simulink model "power_supply_image"  (R2023b)
settings: Solver=ode1  StartTime=0.0  StopTime=time/3  FixedStep=1e-6  RelTol=1e-3
undefined symbols (not defined in the file or in its folder): C1, C2, D1, L1, L2
libraries: spsDiodeLib x13, spsIdealSwitchLib x8, spsVoltageMeasurementLib x6, spsSeriesRLCBranchLib x5, spsCurrentMeasurementLib x2, spsLinearTransformerLib x2, spsDCVoltageSourceLib x1, simulink x1, spspowerguiLib x1
settings Model: Creator=lyapunov  LastModifiedBy=lyapunov
settings OptimizationCC: ReuseModelBlockBuffer=off

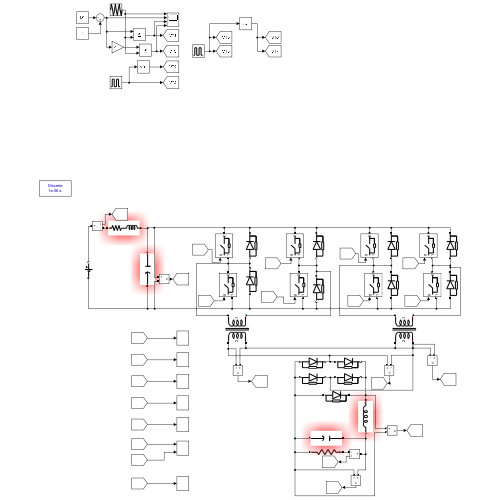
[thumbnail: Simulink's stored preview of the top-level diagram]
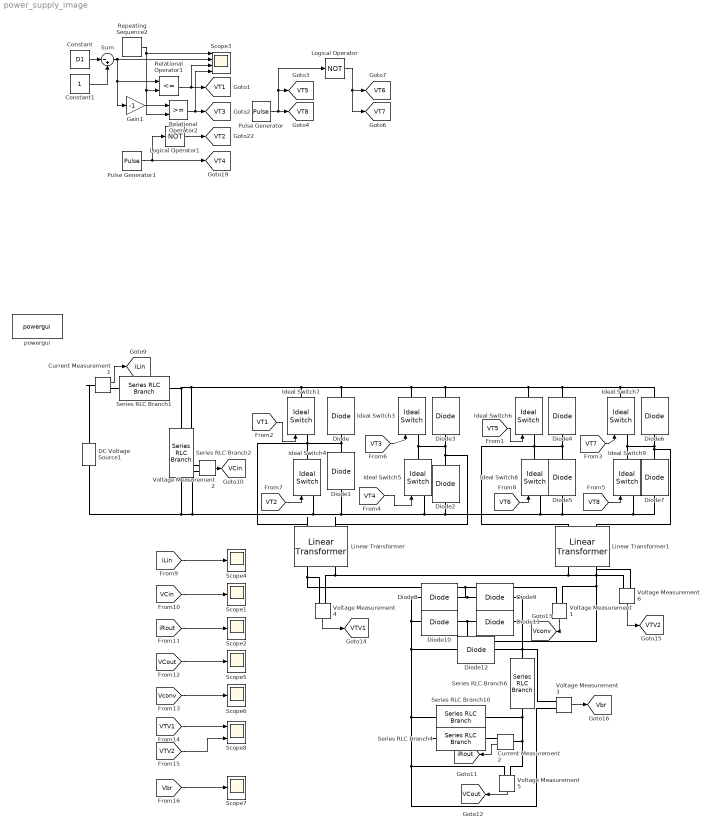
== system power_supply_image ==
  Constant : Constant  Value=D1
  Constant1 : Constant
  Current Measurement1 : spsCurrentMeasurementLib/Current Measurement  PhasorSimulation=off  OutputType=Complex  PSBequivalent=0
  Current Measurement2 : spsCurrentMeasurementLib/Current Measurement  PhasorSimulation=off  OutputType=Complex  PSBequivalent=0
  DC Voltage Source1 : spsDCVoltageSourceLib/DC Voltage Source  Amplitude=300  Measurements=None
  Diode{,1..12} (13 alike) : spsDiodeLib/Diode  Ron=0.001  Lon=0  Vf=0.8  IC=0  UseSnubber=0  Rs=5000  Cs=250e-9  Measurements=off
  Gain1 : Gain  Gain=-1
  Ideal Switch{1,3..9} (8 alike) : spsIdealSwitchLib/Ideal Switch  Ron=0.001  Lon=0  IC=0  Rs=1e5  Cs=inf  Measurements=off
  Linear Transformer : spsLinearTransformerLib/Linear Transformer  UNITS=SI  NominalPower=[500 10000 ]  winding1=[300 0 0]  winding2=[150 0 0]  ThreeWindings=off  winding3=[3.15e+05 0.7938 0.084225]  RmLm=[1e6 1e6]  Measurements=None  DataType=on
  Linear Transformer1 : spsLinearTransformerLib/Linear Transformer  UNITS=SI  NominalPower=[ 500 10000 ]  winding1=[300 0 0]  winding2=[150 0 0]  ThreeWindings=off  winding3=[3.15e+05 0.7938 0.084225]  RmLm=[1e6 1e6]  Measurements=None  DataType=on
  Logical Operator : Logic  Operator=NOT  AllPortsSameDT=off  OutDataTypeStr=boolean
  Logical Operator1 : Logic  Operator=NOT  AllPortsSameDT=off  OutDataTypeStr=boolean
  Pulse Generator : DiscretePulseGenerator  PulseType=Time based  Period=1/10000  PulseWidth=50
  Pulse Generator1 : DiscretePulseGenerator  PulseType=Time based  Period=1/10000  PulseWidth=50
  Relational Operator1 : RelationalOperator  Operator=<=  OutDataTypeStr=boolean  RndMeth=Simplest  InputSameDT=off
  Relational Operator2 : RelationalOperator  OutDataTypeStr=boolean  RndMeth=Simplest  InputSameDT=off
  Repeating Sequence2 : simulink/Sources/Repeating Sequence  rep_seq_t=[0 0.5/20000 1/20000 1.5/20000 2/20000]  rep_seq_y=[0 1 0 -1 0]
  Scope{1..2,4..7} (6 alike) : Scope
  Scope3 : Scope  NumInputPorts=4
  Scope8 : Scope  NumInputPorts=2
  Series RLC Branch1 : spsSeriesRLCBranchLib/Series RLC Branch  LConnTagsString=__new0  RConnTagsString=__new0  BranchType=RL  Resistance=0.01  Inductance=L1  SetiL0=off  InitialCurrent=0  Capacitance=1e-6  Setx0=off  InitialVoltage=0  Measurements=None
  Series RLC Branch10 : spsSeriesRLCBranchLib/Series RLC Branch  LConnTagsString=__new0  RConnTagsString=__new0  BranchType=C  Resistance=1  Inductance=10e-3  SetiL0=off  InitialCurrent=0  Capacitance=C2  Setx0=off  InitialVoltage=0  Measurements=None
  Series RLC Branch2 : spsSeriesRLCBranchLib/Series RLC Branch  LConnTagsString=__new0  RConnTagsString=__new0  BranchType=C  Resistance=1  Inductance=10e-3  SetiL0=off  InitialCurrent=0  Capacitance=C1  Setx0=off  InitialVoltage=0  Measurements=None
  Series RLC Branch4 : spsSeriesRLCBranchLib/Series RLC Branch  LConnTagsString=__new0  RConnTagsString=__new0  BranchType=R  Resistance=87.23  Inductance=10e-3  SetiL0=off  InitialCurrent=0  Capacitance=100e-6  Setx0=off  InitialVoltage=0  Measurements=None
  Series RLC Branch6 : spsSeriesRLCBranchLib/Series RLC Branch  LConnTagsString=__new0  RConnTagsString=__new0  BranchType=L  Resistance=0.01  Inductance=L2  SetiL0=off  InitialCurrent=0  Capacitance=1e-6  Setx0=off  InitialVoltage=0  Measurements=None
  Sum : Sum  Inputs=|-+
  Voltage Measurement{1..6} (6 alike) : spsVoltageMeasurementLib/Voltage Measurement  PhasorSimulation=off  OutputType=Complex  PSBequivalent=0
  powergui : spspowerguiLib/powergui  Priority=1  SimulationMode=Discrete  SampleTime=1e-6  frequency=60  Iterations=50  frequencyindice=0  Pbase=100e6  ErrMax=1e-4  UnitsV=kV  UnitsW=MW  buscounter=0  FunctionMessages=off  echomessages=off  EnableUseOfTLC=off  CurrentSourceSwitches=off  DisableSnubberDevices=off  DisableRonSwitches=off  DisableVfSwitches=off  DisplayEquations=off  AutomaticDiscreteSolvers=off  SolverType=Tustin/Backward Euler (TBE)  Interpol=off  ExternalGateDelay=off  methode=off  Ts=100  x0status=zero  SPID=on  SwTol=0  HookPort=off  NonlinearTolerance=1e-4  nMaxIteration=100  ContinueOnMaxIteration=off  RestoreLinks=warning  ResistiveCurrentMeasurement=off  Frange=[0:2:500]  Ylog=off  Xlog=on  ShowGrid=off  save=off  variable=ZData  structure=0  ZoomFFT=off  StartTime=0.0  cycles=1  DisplayStyle=1  fundamental=60  FreqAxis=off  MaxFrequency=1000  frequencyindicesteady=1  RmsSteady=1  display=off
  tag scope: VCin=global, VCout=global, VT1=global, VT2=global, VT3=global, VT4=global, VT5=global, VT6=global, VT7=global, VT8=global, VTV1=global, VTV2=global, Vbr=global, Vconv=global, iLin=global, iRout=global
  wires:
  Pulse Generator/1 -> Logical Operator/1, [VT5], [VT8]
  Logical Operator/1 -> [VT7], [VT6]
  Repeating Sequence2/1 -> Relational Operator1/2, Relational Operator2/2, Scope3/1
  Relational Operator1/1 -> [VT1], Scope3/3
  Sum/1 -> Relational Operator1/1, Gain1/1, Scope3/2
  Relational Operator2/1 -> [VT3], Scope3/4
  Gain1/1 -> Relational Operator2/1
  [VT5] -> Ideal Switch6/1
  [VT7] -> Ideal Switch7/1
  Constant/1 -> Sum/1
  Constant1/1 -> Sum/2
  Voltage Measurement1/1 -> [Vconv]
  Voltage Measurement2/1 -> [VCin]
  [VT8] -> Ideal Switch9/1
  [VT4] -> Ideal Switch5/1
  [VT1] -> Ideal Switch1/1
  [VT3] -> Ideal Switch3/1
  [VT2] -> Ideal Switch4/1
  [VT6] -> Ideal Switch8/1
  Current Measurement1/1 -> [iLin]
  Current Measurement2/1 -> [iRout]
  Voltage Measurement5/1 -> [VCout]
  [iLin] -> Scope4/1
  [VCin] -> Scope1/1
  [iRout] -> Scope2/1
  [VCout] -> Scope5/1
  [Vconv] -> Scope6/1
  Voltage Measurement3/1 -> [Vbr]
  Voltage Measurement4/1 -> [VTV1]
  Voltage Measurement6/1 -> [VTV2]
  [VTV1] -> Scope8/1
  [VTV2] -> Scope8/2
  [Vbr] -> Scope7/1
  Logical Operator1/1 -> [VT2]
  Pulse Generator1/1 -> Logical Operator1/1, [VT4]
  connections:
  Current Measurement1/RConn1 -- Series RLC Branch1/LConn1
  Current Measurement1/LConn1 -- DC Voltage Source1/RConn1
  Ideal Switch5/RConn1 -- Linear Transformer/LConn1 -- Diode2/RConn1 -- Diode3/LConn1 -- Ideal Switch3/LConn1
  Ideal Switch6/LConn1 -- Ideal Switch8/RConn1 -- Linear Transformer1/LConn2 -- Diode5/RConn1 -- Diode4/LConn1
  Ideal Switch5/LConn1 -- Diode2/LConn1 -- Diode7/LConn1 -- Ideal Switch9/LConn1 -- Diode5/LConn1 -- Ideal Switch8/LConn1 -- Diode1/LConn1 -- DC Voltage Source1/LConn1 -- Series RLC Branch2/RConn1 -- Voltage Measurement2/LConn2 -- Ideal Switch4/LConn1
  Ideal Switch1/LConn1 -- Ideal Switch4/RConn1 -- Linear Transformer/LConn2 -- Diode/LConn1 -- Diode1/RConn1
  Ideal Switch9/RConn1 -- Diode7/RConn1 -- Linear Transformer1/LConn1 -- Diode6/LConn1 -- Ideal Switch7/LConn1
  Diode8/RConn1 -- Voltage Measurement4/LConn2 -- Linear Transformer/RConn2 -- Voltage Measurement1/LConn1 -- Diode9/LConn1
  Linear Transformer1/RConn1 -- Voltage Measurement6/LConn1 -- Diode10/RConn1 -- Diode11/LConn1 -- Voltage Measurement1/LConn2
  Series RLC Branch4/RConn1 -- Voltage Measurement5/LConn2 -- Voltage Measurement3/LConn2 -- Diode12/LConn1 -- Diode8/LConn1 -- Diode10/LConn1 -- Series RLC Branch10/RConn1
  Diode9/RConn1 -- Series RLC Branch6/LConn1 -- Voltage Measurement3/LConn1 -- Diode12/RConn1 -- Diode11/RConn1
  Series RLC Branch10/LConn1 -- Current Measurement2/LConn1 -- Voltage Measurement5/LConn1 -- Series RLC Branch6/RConn1
  Diode4/RConn1 -- Series RLC Branch1/RConn1 -- Series RLC Branch2/LConn1 -- Voltage Measurement2/LConn1 -- Ideal Switch1/RConn1 -- Diode/RConn1 -- Ideal Switch3/RConn1 -- Diode3/RConn1 -- Ideal Switch6/RConn1 -- Diode6/RConn1 -- Ideal Switch7/RConn1
  Current Measurement2/RConn1 -- Series RLC Branch4/LConn1
  Linear Transformer1/RConn2 -- Voltage Measurement6/LConn2 -- Voltage Measurement4/LConn1 -- Linear Transformer/RConn1
